simulink model "Noa_Nofusion"  (R2020b)
settings: Solver=FixedStepDiscrete  StartTime=0.0  StopTime=Inf  FixedStep=0.01  RelTol=1e-3
PostLoadFcn:
  | if any(exist('dsrtsu_mdlpostloadfcn', 'file') ~= 0), dsrtsu_mdlpostloadfcn('Execute', bdroot); end
InitFcn:
  | , if any(exist('rtifpga_mdlclblib', 'file') ~= 0), rtifpga_mdlclblib('Init', bdroot); end,
  | , if any(exist('dsmpb_private', 'file') ~= 0), dsmpb_private('dsmpb_mdlclblib', 'Init', bdroot); end,
undefined symbols (not defined in the file or in its folder): ACC_TimeGap_DecSetSwt, ACC_TimeGap_IncSetSwt, AccelPedalPosn, AccelPedalPosnVldty, AccelPedlPosnDiagc, AccPedalOverride, ACU_ShiftInProgress, ADAS_Posn_CurLane, AESSwtReq, ALC_SwtReq, BrkPedalSts, CC_ACC_CANCEL_OFFSwt, CC_ACC_CRUISE_OFFSwt, CC_ACC_DecSetSpd_SetSwt, CC_ACC_IncSetSpd_ResuSwt, CC_ACCSwtErr, CharSpd_ms, CSA_NODE, CURRENT_GEAR, CurrentGearValid, DiscIntNeverNeededParam, DrvDoorSts, DrvSBR, DrvTrqReqOvld, ECMACCInterface, ECMRespACC, ELKSwtReq, EngLimpHomeSts, EngSpd, EngState, EngState_PHEV, EngTrqMaxActSpd, EngTrqMinAct, EPS_DrvInpTrqVal_HighReslolution, EPS_FailSts, EPS_LKATorqOvrlDlvd, EPS_LKATorqOvrlDlvdVld, EPS_LKATrqOvlDlvdSts, EPS_SteerMod, EPS_TrqSnsrSts, EQ4_APPINFO, EQ4_LA_ELEM, EQ4_LA_HDR, EQ4_LAP_ELEM, EQ4_LAP_HDR, EQ4_LH_ELEM, EQ4_LH_HDR, EQ4_LRE_ELEM, EQ4_LRE_HDR, ESS_PedSwtReq, ESS_VehSwtReq, FFogLmpSts_F_Pbox, FLWheelDriveDirection, FLWheelSpd, FrntWiprSwtSts, FrntWshrSwtSts, FRWheelDriveDirection, FRWheelSpd, HazardLmpSwtSts, HCU_AccelPedalPosn_Diag ... (+151)
libraries: simulink x144, dsmpblib x33, canfdmsglib x10
(part 8 of 20)

== system Noa_Nofusion/TOS2/Subsystem ==
  TOS_ACCP0 : Inport
  Bus Selector : BusSelector  OutputSignals=ACCTgtObjAy,ACCTgtObjCntAlive,ACCTgtObjExist,ACCTgtObjObstcl,ACCTgtObjVy,IDP0,ObjDYP0,ObjMovingStateP0,ObjTypeP0,Object_Orientation,P0CutInflg,P0HeadingAngle,axAbsGroundP0,dxP0,fu_typeP0,rangeP0,targetExistP0,vxRelP0
  CAN FD Pack : canfdmsglib/CAN FD Pack  CANdbFile=F:\InternalData03_ACC_AEBLog_ELK_LC_LCKie_20200927.dbc  MsgList=(none)  MsgName=TOS_ACC_P0  ProtocolMode=CAN FD  MsgIDType=Standard (11-bit identifier)  MsgIdentifier=512  MsgLength=64  Remote=off  BRSSwitch=off  ApplyMinMax=off  SignalInfo={'P0_ACCTgtObjAy','12','12','BE','signed','Standard','0','0.01','0','-20.48','20.47';'P0_ACCTgtObjCntAlive','16','8','BE','unsigned','Standard','0','1','0','0','255';'P0_ACCTgtObjExist','24','8','BE','unsigned','Standard','0','0.01','0','0','2.55';'P0_ACCTgtObjObstcl','46','10','BE','unsigned','Standard','0','0.001','0','0','1.023';'P0_ACCTgtObjVy','58','14','BE','signed','Standard','0','0.01','0','-81.92','81.91';'P0_IDP0','96','8','BE','unsigned','Standard','0','1','0','0','255';'P0_ObjDYP0','114','14','BE','signed','Standard','0','0.005','0','-40.96','40.955';'P0_ObjMovingStateP0','122','6','BE','unsigned','Standard','0','1','0','0','63';'P0_ObjTypeP0','72','4','BE','unsigned','Standard','0','1','0','0','15';'P0_Object_Orientation','8','4','BE','unsigned','Standard','0','1','0','0','15';'P0_P0CutInflg','57','1','BE','unsigned','Standard','0','1','0','0','1';'P0_P0HeadingAngle','128','8','BE','unsigned','Standard','0','0.0041','0','0','1.0455';'P0_axAbsGroundP0','76','12','BE','signed','Standard','0','0.01','0','-20.48','20.47';'P0_dxP0','89','15','BE','unsigned','Standard','0','0.0063','0','0','206.4321';'P0_fu_typeP0','40','6','BE','unsigned','Standard','0','1','0','0','63';'P0_rangeP0','145','15','BE','unsigned','Standard','0','0.01','0','0','327.67';'P0_targetExistP0','56','1','BE','unsigned','Standard','0','1','0','0','1';'P0_vxRelP0','160','16','BE','signed','Standard','0','0.00616','0','-201.8509','201.8447'}
      settings: SourceProductBaseCode=ME,XP,VN  DataFormat=CANdb specified signals
  Out1 : Outport
  wires:
  Bus Selector/4 -> CAN FD Pack/4  "<ACCTgtObjObstcl>"
  Bus Selector/16 -> CAN FD Pack/16  "<rangeP0>"
  Bus Selector/1 -> CAN FD Pack/1  "<ACCTgtObjAy>"
  Bus Selector/8 -> CAN FD Pack/8  "<ObjMovingStateP0>"
  Bus Selector/15 -> CAN FD Pack/15  "<fu_typeP0>"
  Bus Selector/13 -> CAN FD Pack/13  "<axAbsGroundP0>"
  TOS_ACCP0/1 -> Bus Selector/1
  Bus Selector/14 -> CAN FD Pack/14  "<dxP0>"
  Bus Selector/9 -> CAN FD Pack/9  "<ObjTypeP0>"
  Bus Selector/12 -> CAN FD Pack/12  "<P0HeadingAngle>"
  Bus Selector/17 -> CAN FD Pack/17  "<targetExistP0>"
  Bus Selector/5 -> CAN FD Pack/5  "<ACCTgtObjVy>"
  Bus Selector/3 -> CAN FD Pack/3  "<ACCTgtObjExist>"
  Bus Selector/18 -> CAN FD Pack/18  "<vxRelP0>"
  Bus Selector/11 -> CAN FD Pack/11  "<P0CutInflg>"
  Bus Selector/7 -> CAN FD Pack/7  "<ObjDYP0>"
  Bus Selector/2 -> CAN FD Pack/2  "<ACCTgtObjCntAlive>"
  Bus Selector/10 -> CAN FD Pack/10  "<Object_Orientation>"
  Bus Selector/6 -> CAN FD Pack/6  "<IDP0>"
  CAN FD Pack/1 -> Out1/1

== system Noa_Nofusion/TOS2/Subsystem1 ==
  IfStateMBus : Inport
  IfVIEBus : Inport  Port=2
  IfVCAN : Inport  Port=3  OutDataTypeStr=Bus: VCAN_BUS
  visMsg : Inport  Port=4
  function : TriggerPort  TriggerType=function-call  VariantControl=Variant
  ACCOSM : Subsystem
  Bus Selector16 : BusSelector  OutputSignals=VSM_HMI.LCKSts,VSM_LAT_CTRL
  Bus Selector17 : BusSelector  OutputSignals=VSM_LON_CTRL.ACC_TimeGapSet,VSM_LON_CTRL.ACCSts
  Counter Free-Running : simulink/Sources/Counter Free-Running  NumBits=3  tsamp=-1
  Data Type Conversion : DataTypeConversion
  TOS_ACCP0 : Outport  OutDataTypeStr=Bus: TOS_ACCP0_BUS
  TOS_ACCP1 : Outport  Port=2  OutDataTypeStr=Bus: TOS_ACCP1_BUS  PortDimensions=1  BusOutputAsStruct=on
  ACCP2 : Outport  Port=3  OutDataTypeStr=Bus: TOS_ACCP2_BUS
  ACCP3 : Outport  Port=4  OutDataTypeStr=Bus: TOS_ACCP3_BUS
  TOS_ACCP4 : Outport  Port=5  OutDataTypeStr=Bus: TOS_ACCP4_BUS  PortDimensions=1  BusOutputAsStruct=on
  TOS_ACCP5 : Outport  Port=6  OutDataTypeStr=Bus: TOS_ACCP5_BUS  PortDimensions=1  BusOutputAsStruct=on
  TOS_ELK : Outport  Port=7  OutDataTypeStr=Bus: TOS_ELK_BUS  PortDimensions=1  BusOutputAsStruct=on
  TOS_LCKIE : Outport  Port=8  OutDataTypeStr=Bus: TOS_LCKIE_BUS  PortDimensions=1  BusOutputAsStruct=on
  TOS_AEB_LONOBJ : Outport  Port=9  OutDataTypeStr=Bus: TOS_AEB_LONOBJ_BUS  PortDimensions=1  BusOutputAsStruct=on
  TOS_AEB_LATOBJ : Outport  Port=10  OutDataTypeStr=Bus: TOS_AEB_LATOBJ_BUS  PortDimensions=10  BusOutputAsStruct=on
  TOS_AEB_JAOBJ : Outport  Port=11  OutDataTypeStr=Bus: TOS_AEB_JAOBJ_BUS  PortDimensions=32  BusOutputAsStruct=on
  TOS_P0_TARGET_LINE : Outport  Port=12  OutDataTypeStr=Bus: TOS_P0_TARGET_LINE_BUS
  TOS_UpdateCnt : Outport  Port=13  OutDataTypeStr=uint32  PortDimensions=1  BusOutputAsStruct=on
  wires:
  IfVIEBus/1 -> ACCOSM/4(VIE)
  Bus Selector16/1 -> ACCOSM/6(LCKSts)  "<LCKSts>"
  visMsg/1 -> ACCOSM/1(visMsg)
  IfStateMBus/1 -> Bus Selector16/1, Bus Selector17/1
  Bus Selector16/2 -> ACCOSM/7(desLane)  "<VSM_LAT_CTRL>"
  Bus Selector17/2 -> ACCOSM/3(ACCMode)  "<ACCSts>"
  Bus Selector17/1 -> ACCOSM/2(TimeGap)  "<ACC_TimeGapSet>"
  IfVCAN/1 -> ACCOSM/5(VCAN)
  ACCOSM/1(ACCP0) -> TOS_ACCP0/1  "TOS_ACCP0"
  ACCOSM/2(TEM_P0_TARGET_LINE) -> TOS_P0_TARGET_LINE/1  "TOS_P0_TARGET_LINE"
  ACCOSM/3(ACCP2) -> ACCP2/1
  ACCOSM/4(ACCP3) -> ACCP3/1
  Counter Free-Running/1 -> Data Type Conversion/1
  Data Type Conversion/1 -> TOS_UpdateCnt/1

== system Noa_Nofusion/aeb/Subsystem ==
  TOS_AEB_LONOBJ : Inport  OutDataTypeStr=Bus: TOS_AEB_LONOBJ_BUS  PortDimensions=1  BusOutputAsStruct=on
  TOS_AEB_LATOBJ : Inport  Port=2  OutDataTypeStr=Bus: TOS_AEB_LATOBJ_BUS  PortDimensions=10  BusOutputAsStruct=on
  TOS_AEB_JAOBJ : Inport  Port=3  OutDataTypeStr=Bus: TOS_AEB_JAOBJ_BUS  PortDimensions=32  BusOutputAsStruct=on
  vxvRefMs : Inport  Port=4  OutDataTypeStr=single  PortDimensions=1  BusOutputAsStruct=on
  axvRefMs2 : Inport  Port=5  OutDataTypeStr=single  PortDimensions=1  BusOutputAsStruct=on
  ayvRefMs2 : Inport  Port=6  OutDataTypeStr=single  PortDimensions=1  BusOutputAsStruct=on
  kapTraj : Inport  Port=7  OutDataTypeStr=single  PortDimensions=1  BusOutputAsStruct=on
  psiDtOpt : Inport  Port=8  OutDataTypeStr=single  PortDimensions=1  BusOutputAsStruct=on
  AEB_VCAN_ABM : Inport  Port=9  OutDataTypeStr=Bus: AEB_VCAN_ABM_BUS  PortDimensions=1  BusOutputAsStruct=on
  AEB_VCAN_ESP : Inport  Port=10  OutDataTypeStr=Bus: AEB_VCAN_ESP_BUS  PortDimensions=1  BusOutputAsStruct=on
  AEB_VCAN_BCM : Inport  Port=11  OutDataTypeStr=Bus: AEB_VCAN_BCM_BUS  PortDimensions=1  BusOutputAsStruct=on
  AEB_VCAN_CSA : Inport  Port=12  OutDataTypeStr=Bus: AEB_VCAN_CSA_BUS  PortDimensions=1  BusOutputAsStruct=on
  AEB_VCAN_DCT : Inport  Port=13  OutDataTypeStr=Bus: AEB_VCAN_DCT_BUS  PortDimensions=1  BusOutputAsStruct=on
  AEB_VCAN_ECM : Inport  Port=14  OutDataTypeStr=Bus: AEB_VCAN_ECM_BUS  PortDimensions=1  BusOutputAsStruct=on
  AEB_VCAN_HUT : Inport  Port=15  OutDataTypeStr=Bus: AEB_VCAN_HUT_BUS  PortDimensions=1  BusOutputAsStruct=on
  AEB_VCAN_CR : Inport  Port=16  OutDataTypeStr=Bus: AEB_VCAN_CR_BUS  PortDimensions=1  BusOutputAsStruct=on
  AEB_VCAN_HCU : Inport  Port=17  OutDataTypeStr=Bus: AEB_VCAN_HCU_BUS  PortDimensions=1  BusOutputAsStruct=on
  AEB_IB_BrkPedalAppld : Inport  Port=18  OutDataTypeStr=boolean  PortDimensions=1  BusOutputAsStruct=on
  CAL_AEB_CONFIG : Inport  Port=19  OutDataTypeStr=Bus: CAL_AEB_CONFIG_BUS  PortDimensions=1  BusOutputAsStruct=on
  DFIM_AEB_STS : Inport  Port=20  OutDataTypeStr=Bus: DFIM_AEB_STS_BUS  PortDimensions=1  BusOutputAsStruct=on
  VSM_LON_CTRL : Inport  Port=21  OutDataTypeStr=Bus: VSM_LON_CTRL_BUS  PortDimensions=1  BusOutputAsStruct=on
  EQ4_FCF_VD : Inport  Port=22  OutDataTypeStr=Bus: EQ4_FCF_VD_BUS  PortDimensions=1  BusOutputAsStruct=on
  EQ4_FCF_VRU : Inport  Port=23  OutDataTypeStr=Bus: EQ4_FCF_VRU_BUS  PortDimensions=1  BusOutputAsStruct=on
  AEB_BRK_INFO : Outport  OutDataTypeStr=Bus: AEB_BRK_INFO_BUS  PortDimensions=1  BusOutputAsStruct=on
  AEB_DVR_INFO : Outport  Port=2  OutDataTypeStr=Bus: AEB_DVR_INFO_BUS  PortDimensions=1  BusOutputAsStruct=on
  AEB_IPHUT_INFO : Outport  Port=3  OutDataTypeStr=Bus: AEB_IPHUT_INFO_BUS  PortDimensions=1  BusOutputAsStruct=on
  AEB_EDR_LONOBJ_INFO : Outport  Port=4  OutDataTypeStr=Bus: AEB_EDR_LONOBJ_INFO_BUS  PortDimensions=1  BusOutputAsStruct=on
  AEB_EDR_LATPED_INFO : Outport  Port=5  OutDataTypeStr=Bus: AEB_EDR_LATPED_INFO_BUS  PortDimensions=1  BusOutputAsStruct=on
  AEB_EDR_LATCYC_INFO : Outport  Port=6  OutDataTypeStr=Bus: AEB_EDR_LATCYC_INFO_BUS  PortDimensions=1  BusOutputAsStruct=on
  AEB_EDR_JAPED_INFO : Outport  Port=7  OutDataTypeStr=Bus: AEB_EDR_JAPED_INFO_BUS  PortDimensions=1  BusOutputAsStruct=on
  AEB_EDR_JAVEH_INFO : Outport  Port=8  OutDataTypeStr=Bus: AEB_EDR_JAVEH_INFO_BUS  PortDimensions=1  BusOutputAsStruct=on

== system Noa_Nofusion/Chassis1/Subsystem/rollingcounter 1 ==
  Constant7 : Constant  OutDataTypeStr=Inherit: Inherit via back propagation
  Constant8 : Constant  Value=14  OutDataTypeStr=Inherit: Inherit via back propagation
  Constant9 : Constant  Value=0  OutDataTypeStr=Inherit: Inherit via back propagation
  Relational Operator : RelationalOperator  Operator=>  OutDataTypeStr=boolean  RndMeth=Nearest
  Sum : Sum  Inputs=|++
  Switch : Switch  Criteria=u2 ~= 0  Threshold=1
  Unit Delay : UnitDelay  SampleTime=-1  HasFrameUpgradeWarning=on
  cnt : Outport
  wires:
  Switch/1 -> Unit Delay/1, cnt/1
  Relational Operator/1 -> Switch/2
  Constant7/1 -> Sum/1
  Unit Delay/1 -> Sum/2
  Constant8/1 -> Relational Operator/2
  Sum/1 -> Relational Operator/1, Switch/3
  Constant9/1 -> Switch/1

== system Noa_Nofusion/Chassis1/Subsystem/rollingcounter 2 ==
  Constant7 : Constant  OutDataTypeStr=Inherit: Inherit via back propagation
  Constant8 : Constant  Value=14  OutDataTypeStr=Inherit: Inherit via back propagation
  Constant9 : Constant  Value=0  OutDataTypeStr=Inherit: Inherit via back propagation
  Relational Operator : RelationalOperator  Operator=>  OutDataTypeStr=boolean  RndMeth=Nearest
  Sum : Sum  Inputs=|++
  Switch : Switch  Criteria=u2 ~= 0  Threshold=1
  Unit Delay : UnitDelay  SampleTime=-1  HasFrameUpgradeWarning=on
  cnt : Outport
  wires:
  Constant9/1 -> Switch/1
  Sum/1 -> Switch/3, Relational Operator/1
  Constant8/1 -> Relational Operator/2
  Unit Delay/1 -> Sum/2
  Constant7/1 -> Sum/1
  Relational Operator/1 -> Switch/2
  Switch/1 -> cnt/1, Unit Delay/1

== system Noa_Nofusion/Common/Subsystem7/DS ==
  canDMSSts : Inport  OutDataTypeStr=uint8
  canHeadDetn : Inport  Port=2  OutDataTypeStr=boolean
  canDistrctnLevel : Inport  Port=3  OutDataTypeStr=uint8
  canDistrctnQlty : Inport  Port=4  OutDataTypeStr=uint8
  canDrowsnsLevel : Inport  Port=5  OutDataTypeStr=uint8
  DriverStsConditnJudge : Subsystem
  DriverSts_StateMachine : Stateflow chart  TreatAsAtomicUnit=on
  P_DMS_tDSGoodUnbeliv2LowDistrctn : Constant  Value=P_DMS_tDSGoodUnbeliv2LowDistrctn
  P_DMS_tDSGoodUnbeliv2LowDrowsns : Constant  Value=P_DMS_tDSGoodUnbeliv2LowDrowsns
  P_DMS_tDSGoodUnbeliv2MidDistractn : Constant  Value=P_DMS_tDSGoodUnbeliv2MidDistractn
  P_DMS_tDSGoodUnbeliv2MidDrowsns : Constant  Value=P_DMS_tDSGoodUnbeliv2MidDrowsns
  P_DMS_tDSLow2MidDistractn : Constant  Value=P_DMS_tDSLow2MidDistractn
  P_DMS_tDSLow2MidDrowsns : Constant  Value=P_DMS_tDSLow2MidDrowsns
  P_DMS_tDSOther2Hi1Distractn : Constant  Value=P_DMS_tDSOther2Hi1Distractn
  P_DMS_tDSOther2Hi1Drowsns : Constant  Value=P_DMS_tDSOther2Hi1Drowsns
  P_DMS_tDSOther2Hi2Distractn : Constant  Value=P_DMS_tDSOther2Hi2Distractn
  P_DMS_tDSOther2Hi2Drowsns : Constant  Value=P_DMS_tDSOther2Hi2Drowsns
  DistractnSts : Outport  OutDataTypeStr=uint8
  DrowsnsSts : Outport  Port=2  OutDataTypeStr=uint8
  DriverSts : Outport  Port=3  OutDataTypeStr=uint8
  wires:
  canDistrctnLevel/1 -> DriverStsConditnJudge/3(canDistrctnLevel)
  canDistrctnQlty/1 -> DriverStsConditnJudge/4(canDistrctnQlty)
  canHeadDetn/1 -> DriverStsConditnJudge/2(canHeadDetn)
  canDrowsnsLevel/1 -> DriverStsConditnJudge/5(canDrowsnsLevel)
  canDMSSts/1 -> DriverStsConditnJudge/1(canDMSSts)
  P_DMS_tDSGoodUnbeliv2LowDistrctn/1 -> DriverStsConditnJudge/6(PtDSGoodUnbeliv2LowDistrctn)
  P_DMS_tDSGoodUnbeliv2MidDistractn/1 -> DriverStsConditnJudge/7(PtDSGoodUnbeliv2MidDistractn)
  P_DMS_tDSLow2MidDistractn/1 -> DriverStsConditnJudge/8(PtDSLow2MidDistractn)
  P_DMS_tDSOther2Hi1Distractn/1 -> DriverStsConditnJudge/9(PtDSOther2Hi1Distractn)
  P_DMS_tDSOther2Hi2Distractn/1 -> DriverStsConditnJudge/10(PtDSOther2Hi2Distractn)
  P_DMS_tDSGoodUnbeliv2LowDrowsns/1 -> DriverStsConditnJudge/11(PtDSGoodUnbeliv2LowDrowsns)
  P_DMS_tDSGoodUnbeliv2MidDrowsns/1 -> DriverStsConditnJudge/12(PtDSGoodUnbeliv2MidDrowsns)
  P_DMS_tDSLow2MidDrowsns/1 -> DriverStsConditnJudge/13(PtDSLow2MidDrowsns)
  P_DMS_tDSOther2Hi1Drowsns/1 -> DriverStsConditnJudge/14(PtDSOther2Hi1Drowsns)
  P_DMS_tDSOther2Hi2Drowsns/1 -> DriverStsConditnJudge/15(PtDSOther2Hi2Drowsns)
  DriverStsConditnJudge/1(DSOther2Good) -> DriverSts_StateMachine/1(DSOther2Good)
  DriverStsConditnJudge/2(DSOther2Unbeliv) -> DriverSts_StateMachine/2(DSOther2Unbeliv)
  DriverStsConditnJudge/3(DSGoodUnbeliv2LowDistractn) -> DriverSts_StateMachine/3(DSGoodUnbeliv2LowDistractn)
  DriverStsConditnJudge/4(DSMidHi1Hi22LowDistractn) -> DriverSts_StateMachine/4(DSMidHi1Hi22LowDistractn)
  DriverStsConditnJudge/5(DSGoodUnbeliv2MidDistractn) -> DriverSts_StateMachine/5(DSGoodUnbeliv2MidDistractn)
  DriverStsConditnJudge/6(DSLow2MidDistractn) -> DriverSts_StateMachine/6(DSLow2MidDistractn)
  DriverStsConditnJudge/7(DSHi1Hi22MidDistractn) -> DriverSts_StateMachine/7(DSHi1Hi22MidDistractn)
  DriverStsConditnJudge/8(DSOther2Hi1Distractn) -> DriverSts_StateMachine/8(DSOther2Hi1Distractn)
  DriverStsConditnJudge/9(DSOther2Hi2Distractn) -> DriverSts_StateMachine/9(DSOther2Hi2Distractn)
  DriverStsConditnJudge/10(DSGoodUnbeliv2LowDrowsns) -> DriverSts_StateMachine/10(DSGoodUnbeliv2LowDrowsns)
  DriverStsConditnJudge/11(DSMidHi1Hi22LowDrowsns) -> DriverSts_StateMachine/11(DSMidHi1Hi22LowDrowsns)
  DriverStsConditnJudge/12(DSGoodUnbeliv2MidDrowsns) -> DriverSts_StateMachine/12(DSGoodUnbeliv2MidDrowsns)
  DriverStsConditnJudge/13(DSLow2MidDrowsns) -> DriverSts_StateMachine/13(DSLow2MidDrowsns)
  DriverStsConditnJudge/14(DSHi1Hi22MidDrowsns) -> DriverSts_StateMachine/14(DSHi1Hi22MidDrowsns)
  DriverStsConditnJudge/15(DSOther2Hi1Drowsns) -> DriverSts_StateMachine/15(DSOther2Hi1Drowsns)
  DriverStsConditnJudge/16(DSOther2Hi2Drowsns) -> DriverSts_StateMachine/16(DSOther2Hi2Drowsns)
  DriverStsConditnJudge/17(DSMidHi1Hi22NoDistractn) -> DriverSts_StateMachine/17(DSMidHi1Hi22NoDistractn)
  DriverStsConditnJudge/18(DSMidHi1Hi22NoDrowsns) -> DriverSts_StateMachine/18(DSMidHi1Hi22NoDrowsns)
  DriverStsConditnJudge/19(DSUnbeliv2DDAEnable) -> DriverSts_StateMachine/19(DSUnbeliv2DDAEnable)
  DriverSts_StateMachine/1(DistractnSts) -> DistractnSts/1
  DriverSts_StateMachine/2(DrowsnsSts) -> DrowsnsSts/1
  DriverSts_StateMachine/3(DriverSts) -> DriverSts/1

== system Noa_Nofusion/LPV/Subsystem5/For Each Subsystem1 ==
  In1 : Inport  Partition=on  PartitionDimension=1  PartitionWidth=1  PartitionOffset=0
  Bus Assignment4 : BusAssignment  AssignedSignals=LH_CRC,LH_Is_Triggered_SDM_Type,LH_Is_Triggered_SDM_Model,LH_Track_ID,LH_Age,LH_Confidence,Reserved_3,LH_Prediction_Reason,LH_Availability_State,LH_Color,LH_Color_Confidence,LH_Lanemark_Type,LH_DLM_Type,LH_DECEL_Type,Reserved_4,LH_Lanemark_Type_Conf,LH_Side,LH_Crossing,LH_Marker_Width,LH_Marker_Width_STD,Reserved_5,LH_Dash_Average_Length,LH_Dash_Average_Gap,LH_Is_Multi_Clothoid,Reserved_6,LH_Line_First_C0,LH_Line_First_C1,LH_Line_First_C2,LH_Line_First_C3,LH_First_VR_Start,LH_First_VR_End,Reserved_7,LH_First_Measured_VR_End,LH_Second_Measured_VR_End,Reserved_8,LH_Line_Second_C0,LH_Line_Second_C1,LH_Line_Second_C2,LH_Line_Second_C3,LH_Second_VR_Start,LH_Second_VR_End,LH_Buffer_C3
  Bus Selector : BusSelector  OutputSignals=LH_CRC,LH_Is_Triggered_SDM_Type,LH_Is_Triggered_SDM_Model,LH_Track_ID,LH_Age,LH_Confidence,Reserved_3,LH_Prediction_Reason,LH_Availability_State,LH_Color,LH_Color_Confidence,LH_Lanemark_Type,LH_DLM_Type,LH_DECEL_Type,Reserved_4,LH_Lanemark_Type_Conf,LH_Side,LH_Crossing,LH_Marker_Width,LH_Marker_Width_STD,Reserved_5,LH_Dash_Average_Length,LH_Dash_Average_Gap,LH_Is_Multi_Clothoid,Reserved_6,LH_Line_First_C0,LH_Line_First_C1,LH_Line_First_C2,LH_Line_First_C3,LH_First_VR_Start,LH_First_VR_End,Reserved_7,LH_First_Measured_VR_End,LH_Second_Measured_VR_End,Reserved_8,LH_Line_Second_C0,LH_Line_Second_C1,LH_Line_Second_C2,LH_Line_Second_C3,LH_Second_VR_Start,LH_Second_VR_End,LH_Buffer_C3
  Constant4 : Constant  Value=0  OutDataTypeStr=Bus: EQ4_LH_ELEM_BUS
  For Each : ForEach  DisableCoverage=on
  Out1 : Outport  ConcatenationDimension=1
  wires:
  Constant4/1 -> Bus Assignment4/1
  In1/1 -> Bus Selector/1
  Bus Assignment4/1 -> Out1/1
  Bus Selector/1 -> Bus Assignment4/2  "<LH_CRC>"
  Bus Selector/2 -> Bus Assignment4/3  "<LH_Is_Triggered_SDM_Type>"
  Bus Selector/3 -> Bus Assignment4/4  "<LH_Is_Triggered_SDM_Model>"
  Bus Selector/4 -> Bus Assignment4/5  "<LH_Track_ID>"
  Bus Selector/5 -> Bus Assignment4/6  "<LH_Age>"
  Bus Selector/6 -> Bus Assignment4/7  "<LH_Confidence>"
  Bus Selector/7 -> Bus Assignment4/8  "<Reserved_3>"
  Bus Selector/8 -> Bus Assignment4/9  "<LH_Prediction_Reason>"
  Bus Selector/9 -> Bus Assignment4/10  "<LH_Availability_State>"
  Bus Selector/10 -> Bus Assignment4/11  "<LH_Color>"
  Bus Selector/11 -> Bus Assignment4/12  "<LH_Color_Confidence>"
  Bus Selector/12 -> Bus Assignment4/13  "<LH_Lanemark_Type>"
  Bus Selector/13 -> Bus Assignment4/14  "<LH_DLM_Type>"
  Bus Selector/14 -> Bus Assignment4/15  "<LH_DECEL_Type>"
  Bus Selector/15 -> Bus Assignment4/16  "<Reserved_4>"
  Bus Selector/16 -> Bus Assignment4/17  "<LH_Lanemark_Type_Conf>"
  Bus Selector/17 -> Bus Assignment4/18  "<LH_Side>"
  Bus Selector/18 -> Bus Assignment4/19  "<LH_Crossing>"
  Bus Selector/19 -> Bus Assignment4/20  "<LH_Marker_Width>"
  Bus Selector/20 -> Bus Assignment4/21  "<LH_Marker_Width_STD>"
  Bus Selector/21 -> Bus Assignment4/22  "<Reserved_5>"
  Bus Selector/22 -> Bus Assignment4/23  "<LH_Dash_Average_Length>"
  Bus Selector/23 -> Bus Assignment4/24  "<LH_Dash_Average_Gap>"
  Bus Selector/24 -> Bus Assignment4/25  "<LH_Is_Multi_Clothoid>"
  Bus Selector/25 -> Bus Assignment4/26  "<Reserved_6>"
  Bus Selector/26 -> Bus Assignment4/27  "<LH_Line_First_C0>"
  Bus Selector/27 -> Bus Assignment4/28  "<LH_Line_First_C1>"
  Bus Selector/28 -> Bus Assignment4/29  "<LH_Line_First_C2>"
  Bus Selector/29 -> Bus Assignment4/30  "<LH_Line_First_C3>"
  Bus Selector/30 -> Bus Assignment4/31  "<LH_First_VR_Start>"
  Bus Selector/31 -> Bus Assignment4/32  "<LH_First_VR_End>"
  Bus Selector/32 -> Bus Assignment4/33  "<Reserved_7>"
  Bus Selector/33 -> Bus Assignment4/34  "<LH_First_Measured_VR_End>"
  Bus Selector/34 -> Bus Assignment4/35  "<LH_Second_Measured_VR_End>"
  Bus Selector/35 -> Bus Assignment4/36  "<Reserved_8>"
  Bus Selector/36 -> Bus Assignment4/37  "<LH_Line_Second_C0>"
  Bus Selector/37 -> Bus Assignment4/38  "<LH_Line_Second_C1>"
  Bus Selector/38 -> Bus Assignment4/39  "<LH_Line_Second_C2>"
  Bus Selector/39 -> Bus Assignment4/40  "<LH_Line_Second_C3>"
  Bus Selector/40 -> Bus Assignment4/41  "<LH_Second_VR_Start>"
  Bus Selector/41 -> Bus Assignment4/42  "<LH_Second_VR_End>"
  Bus Selector/42 -> Bus Assignment4/43  "<LH_Buffer_C3>"

== system Noa_Nofusion/LPV/Subsystem5/For Each Subsystem2 ==
  In1 : Inport  Partition=on  PartitionDimension=1  PartitionWidth=1  PartitionOffset=0
  Bus Assignment4 : BusAssignment  AssignedSignals=LRE_ID,LRE_Age,LRE_Confidence,LRE_Type,Reserved_2,LRE_Prediction_Reason,LRE_Availability_State,LRE_Height,LRE_Height_STD,Reserved_3,LRE_View_Range_Start,LRE_View_Range_End,Reserved_4,LRE_Measured_VR_End,LRE_Side,LRE_Is_Triggered_SDM_Model,Reserved_5,LRE_Line_C3,LRE_Line_C2,LRE_Line_C1,LRE_Line_C0,LRE_Detection_Source,Reserved_6
  Bus Selector : BusSelector  OutputSignals=LRE_ID,LRE_Age,LRE_Confidence,LRE_Type,Reserved_2,LRE_Prediction_Reason,LRE_Availability_State,LRE_Height,LRE_Height_STD,Reserved_3,LRE_View_Range_Start,LRE_View_Range_End,Reserved_4,LRE_Measured_VR_End,LRE_Side,LRE_Is_Triggered_SDM_Model,Reserved_5,LRE_Line_C3,LRE_Line_C2,LRE_Line_C1,LRE_Line_C0,LRE_Detection_Source,Reserved_6
  Constant4 : Constant  Value=0  OutDataTypeStr=Bus: EQ4_LRE_ELEM_BUS
  For Each : ForEach  DisableCoverage=on
  Out1 : Outport  ConcatenationDimension=1
  wires:
  Bus Assignment4/1 -> Out1/1
  In1/1 -> Bus Selector/1
  Constant4/1 -> Bus Assignment4/1
  Bus Selector/1 -> Bus Assignment4/2  "<LRE_ID>"
  Bus Selector/2 -> Bus Assignment4/3  "<LRE_Age>"
  Bus Selector/3 -> Bus Assignment4/4  "<LRE_Confidence>"
  Bus Selector/4 -> Bus Assignment4/5  "<LRE_Type>"
  Bus Selector/5 -> Bus Assignment4/6  "<Reserved_2>"
  Bus Selector/6 -> Bus Assignment4/7  "<LRE_Prediction_Reason>"
  Bus Selector/7 -> Bus Assignment4/8  "<LRE_Availability_State>"
  Bus Selector/8 -> Bus Assignment4/9  "<LRE_Height>"
  Bus Selector/9 -> Bus Assignment4/10  "<LRE_Height_STD>"
  Bus Selector/10 -> Bus Assignment4/11  "<Reserved_3>"
  Bus Selector/11 -> Bus Assignment4/12  "<LRE_View_Range_Start>"
  Bus Selector/12 -> Bus Assignment4/13  "<LRE_View_Range_End>"
  Bus Selector/13 -> Bus Assignment4/14  "<Reserved_4>"
  Bus Selector/14 -> Bus Assignment4/15  "<LRE_Measured_VR_End>"
  Bus Selector/15 -> Bus Assignment4/16  "<LRE_Side>"
  Bus Selector/16 -> Bus Assignment4/17  "<LRE_Is_Triggered_SDM_Model>"
  Bus Selector/17 -> Bus Assignment4/18  "<Reserved_5>"
  Bus Selector/18 -> Bus Assignment4/19  "<LRE_Line_C3>"
  Bus Selector/19 -> Bus Assignment4/20  "<LRE_Line_C2>"
  Bus Selector/20 -> Bus Assignment4/21  "<LRE_Line_C1>"
  Bus Selector/21 -> Bus Assignment4/22  "<LRE_Line_C0>"
  Bus Selector/22 -> Bus Assignment4/23  "<LRE_Detection_Source>"
  Bus Selector/23 -> Bus Assignment4/24  "<Reserved_6>"

== system Noa_Nofusion/LPV/Subsystem5/For Each Subsystem3 ==
  In1 : Inport  Partition=on  PartitionDimension=1  PartitionWidth=1  PartitionOffset=0
  Bus Assignment4 : BusAssignment  AssignedSignals=LA_Lane_Track_ID,LA_Age,LA_Confidence,LA_Color,LA_Color_Conf,LA_Prediction_Reason,LA_Availability_State,LA_View_Range_Start,Reserved_2,LA_View_Range_End,LA_Measured_VR_End,Reserved_3,LA_Lanemark_Type,LA_DLM_Type,LA_Lanemark_Type_Conf,LA_Line_Side,LA_Marker_Width,Reserved_4,LA_Marker_Width_STD,Reserved_5,LA_Line_C3,LA_Line_C2,LA_Line_C1,LA_Line_C0,LH_Buffer_C1,Reserved_6
  Bus Selector : BusSelector  OutputSignals=LA_Lane_Track_ID,LA_Age,LA_Confidence,LA_Color,LA_Color_Conf,LA_Prediction_Reason,LA_Availability_State,LA_View_Range_Start,Reserved_2,LA_View_Range_End,LA_Measured_VR_End,Reserved_3,LA_Lanemark_Type,LA_DLM_Type,LA_Lanemark_Type_Conf,LA_Line_Side,LA_Marker_Width,Reserved_4,LA_Marker_Width_STD,Reserved_5,LA_Line_C3,LA_Line_C2,LA_Line_C1,LA_Line_C0,LH_Buffer_C1,Reserved_6
  Constant4 : Constant  Value=0  OutDataTypeStr=Bus: EQ4_LA_ELEM_BUS
  For Each : ForEach  DisableCoverage=on
  Out1 : Outport  ConcatenationDimension=1
  wires:
  Bus Assignment4/1 -> Out1/1
  In1/1 -> Bus Selector/1
  Constant4/1 -> Bus Assignment4/1
  Bus Selector/1 -> Bus Assignment4/2  "<LA_Lane_Track_ID>"
  Bus Selector/2 -> Bus Assignment4/3  "<LA_Age>"
  Bus Selector/3 -> Bus Assignment4/4  "<LA_Confidence>"
  Bus Selector/4 -> Bus Assignment4/5  "<LA_Color>"
  Bus Selector/5 -> Bus Assignment4/6  "<LA_Color_Conf>"
  Bus Selector/6 -> Bus Assignment4/7  "<LA_Prediction_Reason>"
  Bus Selector/7 -> Bus Assignment4/8  "<LA_Availability_State>"
  Bus Selector/8 -> Bus Assignment4/9  "<LA_View_Range_Start>"
  Bus Selector/9 -> Bus Assignment4/10  "<Reserved_2>"
  Bus Selector/10 -> Bus Assignment4/11  "<LA_View_Range_End>"
  Bus Selector/11 -> Bus Assignment4/12  "<LA_Measured_VR_End>"
  Bus Selector/12 -> Bus Assignment4/13  "<Reserved_3>"
  Bus Selector/13 -> Bus Assignment4/14  "<LA_Lanemark_Type>"
  Bus Selector/14 -> Bus Assignment4/15  "<LA_DLM_Type>"
  Bus Selector/15 -> Bus Assignment4/16  "<LA_Lanemark_Type_Conf>"
  Bus Selector/16 -> Bus Assignment4/17  "<LA_Line_Side>"
  Bus Selector/17 -> Bus Assignment4/18  "<LA_Marker_Width>"
  Bus Selector/18 -> Bus Assignment4/19  "<Reserved_4>"
  Bus Selector/19 -> Bus Assignment4/20  "<LA_Marker_Width_STD>"
  Bus Selector/20 -> Bus Assignment4/21  "<Reserved_5>"
  Bus Selector/21 -> Bus Assignment4/22  "<LA_Line_C3>"
  Bus Selector/22 -> Bus Assignment4/23  "<LA_Line_C2>"
  Bus Selector/23 -> Bus Assignment4/24  "<LA_Line_C1>"
  Bus Selector/24 -> Bus Assignment4/25  "<LA_Line_C0>"
  Bus Selector/25 -> Bus Assignment4/26  "<LH_Buffer_C1>"
  Bus Selector/26 -> Bus Assignment4/27  "<Reserved_6>"

== system Noa_Nofusion/SimBCM/CSALampCtrlSim/Counter1 ==
  Trigger : Inport
  AND : Logic  AllPortsSameDT=off  OutDataTypeStr=boolean
  Compare To Constant1 : simulink/Logic and Bit Operations/Compare To Constant  relop=>  const=4  OutDataTypeStr=boolean
  Compare To Constant3 : simulink/Logic and Bit Operations/Compare To Constant  relop=<=  const=4  OutDataTypeStr=boolean
  Compare To Constant4 : simulink/Logic and Bit Operations/Compare To Constant  relop=>=  const=1  OutDataTypeStr=boolean
  Constant3 : Constant  OutDataTypeStr=uint16
  Constant4 : Constant  Value=0  OutDataTypeStr=uint16
  Detect Increase : simulink/Logic and Bit Operations/Detect Increase  vinit=0.0  OutDataTypeStr=boolean
  Detect Increase1 : simulink/Logic and Bit Operations/Detect Increase  vinit=0.0  OutDataTypeStr=boolean
  Saturation1 : Saturate  UpperLimit=65000  LowerLimit=0
  Sum : Sum  Inputs=++|
  Switch : Switch  Criteria=u2 ~= 0
  Switch1 : Switch  Criteria=u2 ~= 0
  Unit Delay : UnitDelay  SampleTime=-1  HasFrameUpgradeWarning=on
  Short : Outport
  Long : Outport  Port=2
  wires:
  Detect Increase1/1 -> Long/1
  Detect Increase/1 -> Short/1
  AND/1 -> Detect Increase/1
  Compare To Constant1/1 -> Detect Increase1/1
  Compare To Constant3/1 -> AND/2
  Compare To Constant4/1 -> AND/1
  Saturation1/1 -> Unit Delay/1, Compare To Constant4/1, Compare To Constant3/1, Compare To Constant1/1
  Sum/1 -> Switch1/1
  Trigger/1 -> Switch1/2, Switch/2
  Unit Delay/1 -> Sum/1
  Switch/1 -> Sum/2
  Switch1/1 -> Saturation1/1
  Constant3/1 -> Switch/1
  Constant4/1 -> Switch1/3, Switch/3

== system Noa_Nofusion/SimBCM/CSALampCtrlSim/Counter4 ==
  Trigger : Inport
  AND : Logic  AllPortsSameDT=off  OutDataTypeStr=boolean
  Compare To Constant1 : simulink/Logic and Bit Operations/Compare To Constant  relop=>  const=4  OutDataTypeStr=boolean
  Compare To Constant3 : simulink/Logic and Bit Operations/Compare To Constant  relop=<=  const=4  OutDataTypeStr=boolean
  Compare To Constant4 : simulink/Logic and Bit Operations/Compare To Constant  relop=>=  const=1  OutDataTypeStr=boolean
  Constant3 : Constant  OutDataTypeStr=uint16
  Constant4 : Constant  Value=0  OutDataTypeStr=uint16
  Detect Increase : simulink/Logic and Bit Operations/Detect Increase  vinit=0.0  OutDataTypeStr=boolean
  Detect Increase1 : simulink/Logic and Bit Operations/Detect Increase  vinit=0.0  OutDataTypeStr=boolean
  Saturation1 : Saturate  UpperLimit=65000  LowerLimit=0
  Sum : Sum  Inputs=++|
  Switch : Switch  Criteria=u2 ~= 0
  Switch1 : Switch  Criteria=u2 ~= 0
  Unit Delay : UnitDelay  SampleTime=-1  HasFrameUpgradeWarning=on
  Short : Outport
  Long : Outport  Port=2
  wires:
  Constant4/1 -> Switch/3, Switch1/3
  Constant3/1 -> Switch/1
  Switch1/1 -> Saturation1/1
  Switch/1 -> Sum/2
  Unit Delay/1 -> Sum/1
  Trigger/1 -> Switch/2, Switch1/2
  Sum/1 -> Switch1/1
  Saturation1/1 -> Compare To Constant1/1, Compare To Constant3/1, Compare To Constant4/1, Unit Delay/1
  Compare To Constant4/1 -> AND/1
  Compare To Constant3/1 -> AND/2
  Compare To Constant1/1 -> Detect Increase1/1
  AND/1 -> Detect Increase/1
  Detect Increase/1 -> Short/1
  Detect Increase1/1 -> Long/1

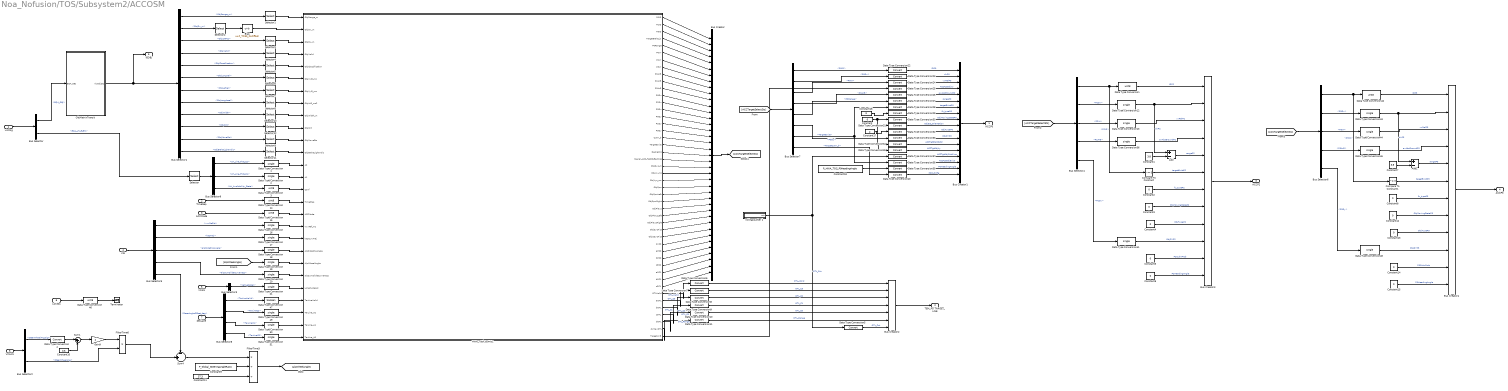
== system Noa_Nofusion/TOS/Subsystem2/ACCOSM ==
  visMsg : Inport
  TimeGap : Inport  Port=2
  ACCMode : Inport  Port=3
  VIE : Inport  Port=4
  VCAN : Inport  Port=5
  LCKSts : Inport  Port=6
  desLane : Inport  Port=7
  Add : Sum  Inputs=+-
  Add1 : Sum  Inputs=+-
  Bias : Bias  Bias=P_TOSS_DxOffset
  Bus Creator : BusCreator  Inputs=39
  Bus Creator1 : BusCreator  Inputs=18  OutDataTypeStr=Bus: TOS_ACCP0_BUS  NonVirtualBus=on
  Bus Creator2 : BusCreator  Inputs=7  OutDataTypeStr=Bus: TOS_P0_TARGET_LINE_BUS  NonVirtualBus=on
  Bus Creator3 : BusCreator  Inputs=12  OutDataTypeStr=Bus: TOS_ACCP2_BUS  NonVirtualBus=on
  Bus Creator4 : BusCreator  Inputs=12  OutDataTypeStr=Bus: TOS_ACCP3_BUS  NonVirtualBus=on
  Bus Selector : BusSelector  OutputSignals=EQ4_OBJ,EQ4_LH.EQ4_LH_ELEM
  Bus Selector4 : BusSelector  OutputSignals=P2ID,P2Dx,P2Vr,P2ArG,P2Dy
  Bus Selector6 : BusSelector  OutputSignals=P3ID,P3Dx,P3Vr,P3ArG,P3Dy
  Bus Selector7 : BusSelector  OutputSignals=P0ID,P0Dx,P0Vr,P0ArG,P0Range,P0Dy,TargetExist,TargetCutIn_b
  Bus Selector9 : BusSelector  OutputSignals=LH_Line_First_C2,LH_Line_First_C1,LH_Availability_State
  Bus Selector1 : BusSelector  OutputSignals=ObjRange_m,ObjDx_m,ObjLatPos,ObjValid,ObjClassification,ObjLongVel,ObjLatVel,ObjLongAccel,ObjWidth,ObjCnt,ObjMoveSts,ObjBrakeLightIndic
  Bus Selector2 : BusSelector  OutputSignals=CSA_NODE.CSA2_MSG.SteerWheelAngSign,CSA_NODE.CSA2_MSG.SteerWheelAng
  Bus Selector3 : BusSelector  OutputSignals=ABM_NODE.ABM2_MSG.VehLgtAccel
  Bus Selector5 : BusSelector  OutputSignals=vxvRefMs,kapTraj,alpSideSlipAngle,alpSumSlideCurveness,SteerAngleOffset_deg
  Bus Selector8 : BusSelector  OutputSignals=TarLineValid,TarLineC2,TarLineC1,TarLineC0
  Compare To Constant : simulink/Logic and Bit Operations/Compare To Constant  relop=~=  const=0  OutDataTypeStr=boolean
  Compare To Constant1 : simulink/Logic and Bit Operations/Compare To Constant  relop=~=  const=0  OutDataTypeStr=boolean
  Constant : Constant  Value=0
  Constant1 : Constant  Value=3.8  OutDataTypeStr=single
  Constant10 : Constant  Value=0.5  OutDataTypeStr=single
  Constant11 : Constant  Value=57.3  OutDataTypeStr=single
  Constant{2..4,8,12..13} (6 alike) : Constant  Value=0  OutDataTypeStr=uint8
  Constant{5..6,14..15} (4 alike) : Constant  Value=0  OutDataTypeStr=single
  Constant16 : Constant  Value=3
  Constant17 : Constant  Value=2
  Constant18 : Constant  Value=P_HWA_TOS_P0HeadingAngle
  Constant7 : Constant  Value=3.8  OutDataTypeStr=single
  Constant9 : Constant  Value=P_Global_SteeringAngleRatio
  Data Type Conversion{,3,14..15,42,46} (6 alike) : DataTypeConversion  OutDataTypeStr=uint8
  Data Type Conversion{1..2,12..13,16..21,36,41,43..45,48..51} (19 alike) : DataTypeConversion  OutDataTypeStr=single
  Data Type Conversion{4..11,22..35,37..40} (26 alike) : DataTypeConversion
  Data Type Conversion47 : DataTypeConversion  OutDataTypeStr=boolean
  FilterTime3 : Product  Inputs=*//  RndMeth=Zero
  FilterTime6 : Product  Inputs=**  RndMeth=Zero
  Gain9 : Gain  Gain=2
  HWA_Task100ms1 : Subsystem
  ObjMatrixTransit : Subsystem
  Selector : Selector  InputPortWidth=2  IndexOptions=Index vector (dialog)  Indices=1  OutputSizes=1
  Selector{1..12} (12 alike) : Selector  InputPortWidth=20  IndexOptions=Index vector (dialog)  Indices=[1:15]  OutputSizes=1
  Sum1 : Sum  Inputs=|-+
  Sum4 : Sum  Inputs=-+|
  Terminator : Terminator
  VCAN1 : InportShadow  Port=5
  rollingcounter 1 : Subsystem
  ACCP0 : Outport  OutDataTypeStr=Bus: TOS_ACCP0_BUS
  TEM_P0_TARGET_LINE : Outport  Port=2  OutDataTypeStr=Bus: TOS_P0_TARGET_LINE_BUS  PortDimensions=1  BusOutputAsStruct=on
  ACCP2 : Outport  Port=3  OutDataTypeStr=Bus: TOS_ACCP2_BUS
  ACCP3 : Outport  Port=4  OutDataTypeStr=Bus: TOS_ACCP3_BUS
  IEOBJ : Outport  Port=5
  wires:
  Bus Creator1/1 -> ACCP0/1
  Bus Selector8/4 -> Data Type Conversion51/1  "<TarLineC0>"
  Data Type Conversion20/1 -> HWA_Task100ms1/22(alpSumSlideCurveness)
  HWA_Task100ms1/23(ObjVy_ms) -> Bus Creator/23
  Data Type Conversion15/1 -> HWA_Task100ms1/17(ACCMode)
  Bus Selector7/7 -> Data Type Conversion28/1, Data Type Conversion38/1  "<TargetExist>"
  HWA_Task100ms1/6(P0Vr) -> Bus Creator/6
  HWA_Task100ms1/25(ObjSpw) -> Bus Creator/25
  [alpWheelAngle] -> Data Type Conversion19/1
  Bus Selector9/3 -> Data Type Conversion3/1  "<LH_Availability_State>"
  desLane/1 -> Bus Selector8/1
  Data Type Conversion40/1 -> Bus Creator1/18  "P0CutInflg"
  HWA_Task100ms1/29(ObjPlausLeft) -> Bus Creator/29
  HWA_Task100ms1/7(P2Vr) -> Bus Creator/7
  Bus Selector1/4 -> Selector4/1  "<ObjValid>"
  Bus Selector8/2 -> Data Type Conversion49/1  "<TarLineC2>"
  Data Type Conversion24/1 -> Bus Creator1/3  "vxRelP0"
  LCKSts/1 -> Data Type Conversion46/1
  HWA_Task100ms1/28(ObjPlaus) -> Bus Creator/28
  Bus Selector1/2 -> Selector2/1  "<ObjDx_m>"
  Data Type Conversion26/1 -> Bus Creator1/5  "axAbsGroundP0"
  HWA_Task100ms1/5(P0Range) -> Bus Creator/5
  HWA_Task100ms1/37(aPC1) -> Bus Creator/37
  HWA_Task100ms1/26(ObjSpwLeft) -> Bus Creator/26
  HWA_Task100ms1/10(P2ArG) -> Bus Creator/10
  Bus Selector1/10 -> Selector12/1  "<ObjCnt>"
  HWA_Task100ms1/19(TargetExist) -> Bus Creator/19
  HWA_Task100ms1/17(P3Dy) -> Bus Creator/17
  HWA_Task100ms1/12(P0Dx) -> Bus Creator/12
  HWA_Task100ms1/39(cPC1) -> Bus Creator/39
  HWA_Task100ms1/36(cPC0) -> Bus Creator/36
  HWA_Task100ms1/9(P0ArG) -> Bus Creator/9
  Bus Selector5/4 -> Data Type Conversion20/1  "<alpSumSlideCurveness>"
  Data Type Conversion33/1 -> Bus Creator1/12  "ObjDYP0"
  HWA_Task100ms1/14(P3Dx) -> Bus Creator/14
  Bus Selector5/3 -> Data Type Conversion18/1  "<alpSideSlipAngle>"
  Bus Selector1/12 -> Selector11/1  "<ObjBrakeLightIndic>"
  Bus Selector1/6 -> Selector6/1  "<ObjLongVel>"
  Bus Selector1/1 -> Selector1/1  "<ObjRange_m>"
  Data Type Conversion50/1 -> HWA_Task100ms1/26(TarLine_A1)
  Data Type Conversion31/1 -> Bus Creator1/10  "Object_Orientation"
  Bus Selector7/4 -> Data Type Conversion26/1  "<P0ArG>"
  HWA_Task100ms1/20(DesireDis) -> Bus Creator/20
  HWA_Task100ms1/3(P3ID) -> Bus Creator/3
  [ACCTargetSelectSts] -> Bus Selector7/1
  HWA_Task100ms1/27(ObjSpwRight) -> Bus Creator/27
  HWA_Task100ms1/18(CutIn_b) -> Bus Creator/18
  Bus Selector9/2 -> Data Type Conversion2/1  "<LH_Line_First_C1>"
  Data Type Conversion16/1 -> HWA_Task100ms1/18(VxvRef_ms)
  HWA_Task100ms1/35(bPC0) -> Bus Creator/35
  Bus Selector1/11 -> Selector9/1  "<ObjMoveSts>"
  HWA_Task100ms1/13(P2Dx) -> Bus Creator/13
  HWA_Task100ms1/30(ObjPlausRight) -> Bus Creator/30
  Bus Selector8/3 -> Data Type Conversion50/1  "<TarLineC1>"
  HWA_Task100ms1/16(P2Dy) -> Bus Creator/16
  HWA_Task100ms1/24(ObjVyc_ms) -> Bus Creator/24
  HWA_Task100ms1/21(Signal_ACC_TgtObjBarDisp) -> Bus Creator/21
  Data Type Conversion39/1 -> Bus Creator1/17  "P0HeadingAngle"
  HWA_Task100ms1/33(dxC0) -> Bus Creator/33
  HWA_Task100ms1/15(P0Dy) -> Bus Creator/15
  Data Type Conversion14/1 -> HWA_Task100ms1/16(TimeGap)
  HWA_Task100ms1/4(TargetBrake_b) -> Bus Creator/4
  Data Type Conversion47/1 -> HWA_Task100ms1/24(TarLineValid)
  Constant/1 -> Data Type Conversion35/1, Data Type Conversion34/1, Data Type Conversion31/1, Data Type Conversion30/1
  Bus Selector1/3 -> Selector3/1  "<ObjLatPos>"
  Bus Selector5/2 -> Data Type Conversion17/1  "<kapTraj>"
  Bus Selector7/5 -> Data Type Conversion27/1  "<P0Range>"
  Bus Selector1/5 -> Selector5/1  "<ObjClassification>"
  HWA_Task100ms1/31(ObjDycHist) -> Bus Creator/31
  Bus Creator/1 -> [ACCTargetSelectSts]
  Data Type Conversion21/1 -> HWA_Task100ms1/23(LongitudeAcc)
  Data Type Conversion23/1 -> Bus Creator1/2  "dxP0"
  TimeGap/1 -> Data Type Conversion14/1
  Data Type Conversion25/1 -> Bus Creator1/4  "ACCTgtObjVy"
  HWA_Task100ms1/11(P3ArG) -> Bus Creator/11
  Data Type Conversion30/1 -> Bus Creator1/9  "ObjMovingStateP0"
  Data Type Conversion18/1 -> HWA_Task100ms1/20(AlpSideSlipAngle)
  HWA_Task100ms1/22(ObjDyc_m) -> Bus Creator/22
  ACCMode/1 -> Data Type Conversion15/1
  Data Type Conversion49/1 -> HWA_Task100ms1/25(TarLine_A2)
  Bus Selector1/8 -> Selector8/1  "<ObjLongAccel>"
  HWA_Task100ms1/8(P3Vr) -> Bus Creator/8
  Bus Selector1/7 -> Selector7/1  "<ObjLatVel>"
  Data Type Conversion28/1 -> Bus Creator1/7  "targetExistP0"
  Data Type Conversion17/1 -> HWA_Task100ms1/19(kapCurvTraj)
  Bus Selector5/1 -> Data Type Conversion16/1  "<vxvRefMs>"
  Bus Selector8/1 -> Data Type Conversion47/1  "<TarLineValid>"
  Data Type Conversion34/1 -> Bus Creator1/13  "ACCTgtObjObstcl"
  VCAN/1 -> Bus Selector3/1
  Data Type Conversion35/1 -> Bus Creator1/14  "ACCTgtObjAy"
  Data Type Conversion32/1 -> Bus Creator1/11  "ObjTypeP0"
  HWA_Task100ms1/32(ObjqDycHist) -> Bus Creator/32
  Bus Selector7/8 -> Data Type Conversion40/1  "<TargetCutIn_b>"
  Data Type Conversion29/1 -> Bus Creator1/8  "fu_typeP0"
  Bus Selector7/2 -> Data Type Conversion23/1  "<P0Dx>"
  Bus Selector7/6 -> Data Type Conversion33/1  "<P0Dy>"
  Data Type Conversion38/1 -> Bus Creator1/16  "ACCTgtObjExist"
  VIE/1 -> Bus Selector5/1
  Bus Selector9/1 -> Data Type Conversion1/1  "<LH_Line_First_C2>"
  Bus Selector7/3 -> Data Type Conversion24/1  "<P0Vr>"
  Data Type Conversion19/1 -> HWA_Task100ms1/21(AlpWheelAngle)
  Bus Selector1/9 -> Selector10/1  "<ObjWidth>"
  Bus Selector3/1 -> Data Type Conversion21/1  "<VehLgtAccel>"
  HWA_Task100ms1/1(P0ID) -> Bus Creator/1
  Data Type Conversion37/1 -> Bus Creator1/15  "ACCTgtObjCntAlive"
  Data Type Conversion2/1 -> HWA_Task100ms1/14(A1)
  HWA_Task100ms1/2(P2ID) -> Bus Creator/2
  Data Type Conversion1/1 -> HWA_Task100ms1/13(A2)
  Data Type Conversion27/1 -> Bus Creator1/6  "rangeP0"
  Data Type Conversion22/1 -> Bus Creator1/1  "IDP0"
  Data Type Conversion3/1 -> HWA_Task100ms1/15(Conf)
  Bus Selector7/1 -> Data Type Conversion22/1  "<P0ID>"
  HWA_Task100ms1/38(bPC1) -> Bus Creator/38
  HWA_Task100ms1/34(aPC0) -> Bus Creator/34
  FilterTime6/1 -> Sum4/2
  Constant11/1 -> FilterTime3/3
  Sum4/1 -> FilterTime3/1
  FilterTime3/1 -> [alpWheelAngle]
  Bus Selector5/5 -> Sum4/1  "<SteerAngleOffset_deg>"
  Constant9/1 -> FilterTime3/2
  VCAN1/1 -> Bus Selector2/1
  Constant10/1 -> Sum1/2
  Gain9/1 -> FilterTime6/1
  Sum1/1 -> Gain9/1
  Bus Selector2/1 -> Data Type Conversion4/1  "<SteerWheelAngSign>"
  Bus Selector2/2 -> FilterTime6/2  "<SteerWheelAng>"
  Data Type Conversion4/1 -> Sum1/1
  HWA_Task100ms1/44(dOTL) -> Data Type Conversion10/1  "OTL_C0"
  HWA_Task100ms1/45(dxMaxOTL) -> Data Type Conversion11/1  "OTL_Range"
  rollingcounter 1/1(cnt) -> Data Type Conversion37/1, Data Type Conversion5/1  "OTL_Cnt"
  HWA_Task100ms1/43(cOTL) -> Data Type Conversion9/1  "OTL_C1"
  HWA_Task100ms1/40(OTLValid) -> Data Type Conversion6/1  "OTL_Valid"
  HWA_Task100ms1/41(aOTL) -> Data Type Conversion7/1  "OTL_C3"
  HWA_Task100ms1/42(bOTL) -> Data Type Conversion8/1  "OTL_C2"
  Bus Creator2/1 -> TEM_P0_TARGET_LINE/1
  Data Type Conversion5/1 -> Bus Creator2/7  "OTL_Cnt"
  Data Type Conversion6/1 -> Bus Creator2/1  "OTL_Valid"
  Data Type Conversion7/1 -> Bus Creator2/2  "OTL_C3"
  Data Type Conversion8/1 -> Bus Creator2/3  "OTL_C2"
  Data Type Conversion9/1 -> Bus Creator2/4  "OTL_C1"
  Data Type Conversion10/1 -> Bus Creator2/5  "OTL_C0"
  Data Type Conversion11/1 -> Bus Creator2/6  "OTL_Range"
  visMsg/1 -> Bus Selector/1
  Bus Selector/2 -> Selector/1  "<EQ4_LH_ELEM>"
  Selector/1 -> Bus Selector9/1
  Selector1/1 -> HWA_Task100ms1/1(ObjRange_m)
  Bias/1 -> HWA_Task100ms1/2(ObjDx_m)
  Selector3/1 -> HWA_Task100ms1/3(ObjDy_m)
  Selector4/1 -> HWA_Task100ms1/4(ObjValid)
  Selector5/1 -> HWA_Task100ms1/5(ObjClassification)
  Selector6/1 -> HWA_Task100ms1/6(ObjVxG_ms)
  Selector7/1 -> HWA_Task100ms1/7(ObjVyG_ms)
  Selector8/1 -> HWA_Task100ms1/8(ObjArG_ms2)
  Selector9/1 -> HWA_Task100ms1/11(ObjMoveSts)
  Selector10/1 -> HWA_Task100ms1/9(ObjWidth_m)
  Selector11/1 -> HWA_Task100ms1/12(ObjBrakeLightIndic)
  Selector12/1 -> HWA_Task100ms1/10(ObjCnt)
  Bus Selector/1 -> ObjMatrixTransit/1(EQ4_OBJ)  "<EQ4_OBJ>"
  ObjMatrixTransit/1(VisObjSts) -> IEOBJ/1, Bus Selector1/1
  [ACCTargetSelectSts] -> Bus Selector4/1
  Bus Selector4/1 -> Compare To Constant/1, Data Type Conversion/1  "<P2ID>"
  Data Type Conversion/1 -> Bus Creator3/1  "IDP2"
  Bus Selector4/2 -> Data Type Conversion12/1  "<P2Dx>"
  Data Type Conversion12/1 -> Add/1, Bus Creator3/2  "dxP2"
  Bus Selector4/3 -> Data Type Conversion13/1  "<P2Vr>"
  Data Type Conversion13/1 -> Bus Creator3/3  "vxRelP2"
  Bus Selector4/4 -> Data Type Conversion36/1  "<P2ArG>"
  Data Type Conversion36/1 -> Bus Creator3/4  "axAbsGroundP2"
  Add/1 -> Bus Creator3/5  "rangeP2"
  Constant1/1 -> Add/2
  Compare To Constant/1 -> Bus Creator3/6  "targetExistP2"
  Constant2/1 -> Bus Creator3/7  "fu_typeP2"
  Constant3/1 -> Bus Creator3/8  "ObjMovingStateP2"
  Constant4/1 -> Bus Creator3/9  "ObjTypeP2"
  Bus Selector4/5 -> Data Type Conversion41/1  "<P2Dy>"
  Data Type Conversion41/1 -> Bus Creator3/10  "ObjDYP2"
  Constant5/1 -> Bus Creator3/11  "P2CutinProb"
  Constant6/1 -> Bus Creator3/12  "P2HeadingAngle"
  Bus Creator3/1 -> ACCP2/1
  Bus Creator4/1 -> ACCP3/1
  Constant15/1 -> Bus Creator4/12  "P3HeadingAngle"
  Constant14/1 -> Bus Creator4/11  "P3CutinProb"
  Data Type Conversion48/1 -> Bus Creator4/10  "ObjDYP3"
  Bus Selector6/5 -> Data Type Conversion48/1  "<P3Dy>"
  Constant13/1 -> Bus Creator4/9  "ObjTypeP3"
  Constant12/1 -> Bus Creator4/8  "ObjMovingStateP3"
  Constant8/1 -> Bus Creator4/7  "fu_typeP3"
  Compare To Constant1/1 -> Bus Creator4/6  "targetExistP3"
  Constant7/1 -> Add1/2
  Add1/1 -> Bus Creator4/5  "rangeP3"
  Data Type Conversion45/1 -> Bus Creator4/4  "axAbsGroundP3"
  Bus Selector6/4 -> Data Type Conversion45/1  "<P3ArG>"
  Data Type Conversion44/1 -> Bus Creator4/3  "vxRelP3"
  Bus Selector6/3 -> Data Type Conversion44/1  "<P3Vr>"
  Data Type Conversion43/1 -> Bus Creator4/2, Add1/1  "dxP3"
  Bus Selector6/2 -> Data Type Conversion43/1  "<P3Dx>"
  Data Type Conversion42/1 -> Bus Creator4/1  "IDP3"
  Bus Selector6/1 -> Data Type Conversion42/1, Compare To Constant1/1  "<P3ID>"
  [ACCTargetSelectSts] -> Bus Selector6/1
  Selector2/1 -> Bias/1
  Constant16/1 -> Data Type Conversion29/1
  Constant17/1 -> Data Type Conversion32/1
  HWA_Task100ms1/46(TargetVyG) -> Data Type Conversion25/1
  Constant18/1 -> Data Type Conversion39/1
  Data Type Conversion46/1 -> Terminator/1
  Data Type Conversion51/1 -> HWA_Task100ms1/27(TarLine_A0)
